simulink model "mcb_bldc_sixstep_f28069mLaunchPad_openLoop"  (R2023b)
settings: Solver=FixedStepDiscrete  StartTime=0.0  StopTime=2  RelTol=1e-3  EnableMultiTasking=on
InitFcn:
  | mcb_bldc_sixstep_f28069mLaunchPad_data;
undefined symbols (not defined in the file): bldc, Down, GPTRIP1SEL, GPTRIP2SEL, target, TZ1, TZ2, Up
libraries: c2806xlib x4, c2802xlib x4, mcbpositiondecoderlib x3, mcbcontrolslib x2, c280xlib x2, simulink x1, svdschedulerlib x1
settings Model: SILPILSystemUnderTest=refmodels  ExtModeTrigDuration=8  VariantFading=off  Creator=The MathWorks, Inc.  LastModifiedBy=Tefilus
settings SolverCC: AlgebraicLoopSolver=TrustRegion  AutoInsertRateTranBlk=on
settings DataIOCC: LimitDataPoints=on  SaveFormat=Array  SaveOutput=off  SaveTime=off  ReturnWorkspaceOutputs=off
settings OptimizationCC: DefaultParameterBehavior=Inlined  DefaultUnderspecifiedDataType=single  OptimizeBlockIOStorage=off  BufferReuse=off  ReuseModelBlockBuffer=off  GlobalBufferReuse=off  ExpressionFolding=off  ExpressionDepthLimit=2147483647  LocalBlockOutputs=off  InitFltsAndDblsToZero=on  NoFixptDivByZeroProtection=on  EfficientFloat2IntCast=on  EfficientMapNaN2IntZero=off  LifeSpan=inf  MaxStackSize=1024  OptimizeDataStoreBuffers=off  BusAssignmentInplaceUpdate=off  DenormalBehavior=FlushToZero  EfficientTunableParamExpr=on
settings DebuggingCC: AlgebraicLoopMsg=error  ArtificialAlgebraicLoopMsg=error  CheckSSInitialOutputMsg=off  MergeDetectMultiDrivingBlocksExec=none  SolverPrmCheckMsg=warning  InheritedTsInSrcMsg=none  MultiTaskDSMMsg=none  MultiTaskCondExecSysMsg=none  TasksWithSamePriorityMsg=none  SigSpecEnsureSampleTimeMsg=none  ParameterPrecisionLossMsg=none  ParameterTunabilityLossMsg=error  FcnCallInpInsideContextMsg=warning  UnconnectedInputMsg=warning  UnconnectedOutputMsg=warning  UnconnectedLineMsg=warning  AllowSymbolicDim=off  StateNameClashWarn=warning  SFUnexpectedBacktrackingDiag=warning  SFNoUnconditionalDefaultTransitionDiag=warning  SFExecutionAtInitializationDiag=none  ArithmeticOperatorsInVariantConditions=warning
settings HardwareCC: ProdBitPerChar=16  ProdBitPerInt=16  ProdBitPerPointer=32  ProdBitPerSizeT=32  ProdBitPerPtrDiffT=32  ProdLargestAtomicInteger=Integer  ProdLargestAtomicFloat=None  ProdWordSize=16  ProdLongLongMode=on  ProdHWDeviceType=Texas Instruments->C2000  TargetBitPerChar=16  TargetBitPerInt=16  TargetLargestAtomicInteger=Integer  TargetLongLongMode=on  TargetIntDivRoundTo=Zero  TargetEndianess=LittleEndian  TargetWordSize=16  TargetHWDeviceType=Texas Instruments->C2000  ProdEqTarget=off
settings ModelReferenceCC: EnableRefExpFcnMdlSchedulingChecks=on  PropagateSignalLabelsOutOfModel=off
settings SFSimCC: SimUseLocalCustomCode=off  MATLABDynamicMemAlloc=off
settings RTWCC: Description=Embedded Coder  SystemTargetFile=ert.tlc  HardwareBoard=TI Piccolo F28069M LaunchPad  TemplateMakefile=ert_default_tmf  PostCodeGenCommand=; codertarget.postCodeGenHookCommand(h)  GenerateReport=on  RTWUseLocalCustomCode=off  Toolchain=Texas Instruments Code Composer Studio (C2000)  IncludeHyperlinkInReport=on  GenerateTraceInfo=on  GenerateTraceReport=on  GenerateTraceReportSl=on  GenerateTraceReportSf=on  GenerateTraceReportEml=on  DLArmComputeVersion=19.05
settings CodeAppCC: IgnoreCustomStorageClasses=off  CustomSymbolStrType=$N$R$M  StateflowObjectComments=on  InternalIdentifier=Classic
settings ERTTargetCC: TargetFcnLib=ansi_tfl_tmw_new.mat  CodeReplacementLibrary=TI C28x  MultiwordLength=2048  ParMdlRefBuildCompliant=off  CompOptLevelCompliant=off  ConcurrentExecutionCompliant=off  CPPClassGenCompliant=off  ExtModeStaticAllocSize=2000  ExtModeMexFile=TIC2000ExternalModeOpen  ExtModeIntrfLevel=Level2 - Open  ConvertIfToSwitch=off  SuppressUnreachableDefaultCases=off  MemSecPackage=tic2000demospkg
settings ConfigComp: CovMetricSettings=dw  CovSaveCumulativeToWorkspaceVar=on  CovSaveSingleToWorkspaceVar=on  CovExternalEMLEnable=off  CovSFcnEnable=off

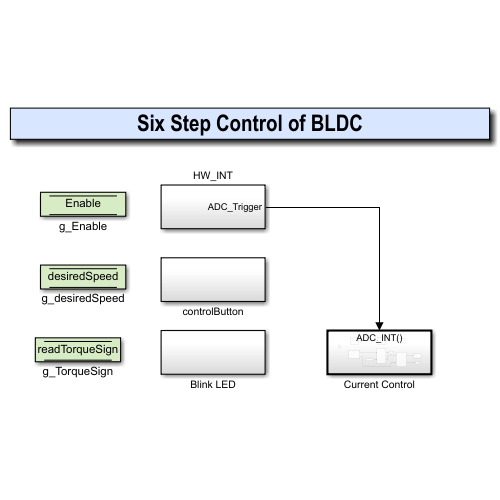
[thumbnail: Simulink's stored preview of the top-level diagram]
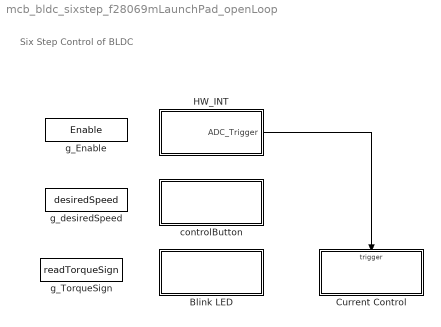
== system mcb_bldc_sixstep_f28069mLaunchPad_openLoop ==
  note: Six Step Control of BLDC
  Blink LED : Subsystem
  Current Control : Subsystem  TreatAsAtomicUnit=on
  HW_INT : Subsystem
  controlButton : Subsystem
  g_Enable : DataStoreMemory  DataStoreName=Enable  ShowAdditionalParam=off  OutDataTypeStr=boolean
  g_TorqueSign : DataStoreMemory  DataStoreName=readTorqueSign  ShowAdditionalParam=off  OutDataTypeStr=boolean
  g_desiredSpeed : DataStoreMemory  DataStoreName=desiredSpeed  ShowAdditionalParam=off
  wires:
  HW_INT/1(ADC_Trigger) -> Current Control/Trigger

== system mcb_bldc_sixstep_f28069mLaunchPad_openLoop/Blink LED ==
  Constant : Constant  SampleTime=0.5
  Digital Output : c2806xlib/Digital Output  GPIO_Number=GPIO32~GPIO39  GPIO_Bit0=off  GPIO_BIT0_Toggle=off  GPIO_Bit1=off  GPIO_BIT1_Toggle=off  GPIO_Bit2=off  GPIO_BIT2_Toggle=off  GPIO_Bit3=off  GPIO_BIT3_Toggle=off  GPIO_Bit4=off  GPIO_BIT4_Toggle=off  GPIO_Bit5=off  GPIO_BIT5_Toggle=off  GPIO_Bit6=off  GPIO_BIT6_Toggle=off  GPIO_Bit7=on  GPIO_BIT7_Toggle=on
  wires:
  Constant/1 -> Digital Output/1

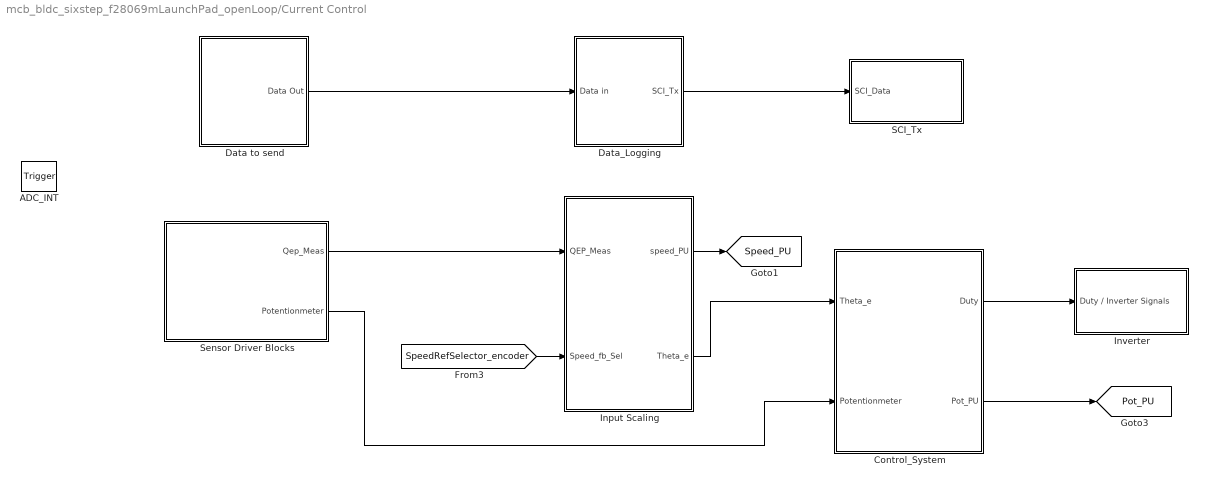
== system mcb_bldc_sixstep_f28069mLaunchPad_openLoop/Current Control ==
  ADC_INT : TriggerPort  TriggerType=function-call  VariantControl=(inherit)
  Control_System : Subsystem
  Data to send : Subsystem
  Data_Logging : Subsystem
  Input Scaling : Subsystem
  Inverter : Subsystem  VariantControl=(codegen)
  SCI_Tx : Subsystem  VariantControl=(codegen)
  Sensor Driver Blocks : Subsystem  VariantControl=(codegen)
  tag scope: Pot_PU=global, Speed_PU=global
  wires:
  Control_System/1(Duty) -> Inverter/1(Duty / Inverter Signals)
  Input Scaling/2(Theta_e) -> Control_System/1(Theta_e)
  Sensor Driver Blocks/2(Potentionmeter) -> Control_System/2(Potentionmeter)
  Data_Logging/1(SCI_Tx) -> SCI_Tx/1(SCI_Data)
  Control_System/2(Pot_PU) -> [Pot_PU]
  Input Scaling/1(speed_PU) -> [Speed_PU]
  [SpeedRefSelector_encoder] -> Input Scaling/2(Speed_fb_Sel)
  Data to send/1(Data Out) -> Data_Logging/1(Data in)
  Sensor Driver Blocks/1(Qep_Meas) -> Input Scaling/1(QEP_Meas)

== system mcb_bldc_sixstep_f28069mLaunchPad_openLoop/HW_INT ==
  HWI_ADCINT1 : svdschedulerlib/Hardware Interrupt v2  ISRGroup=ADC - Analog to Digital Converter  ISRName=ADCA1_INT  ISRNumber=32  NumEventsToServe=1  EventsList={'on','EOC event','1';'off','Overflow event','2';'off','Custom event','3'}  SelectedEvents={'event1'}  TaskPriority=30  DisablePreemption=on  ClearInterruptFlagsAtEndOfEvent=on  InterruptDefinitionFile=$(TARGET_ROOT)/registry/interrupts/F2837xS_interrupts.xml  HardwareBoard=F2837x  EnableSimPort=off
      settings: LibrarySourceBlock=c2000lib/Scheduling/Hardware Interrupt
  ADC_Trigger : Outport
  wires:
  HWI_ADCINT1/1 -> ADC_Trigger/1

== system mcb_bldc_sixstep_f28069mLaunchPad_openLoop/controlButton ==
  CW/CCW_GPIO7 : c2806xlib/Digital Input  GPIO_Number=GPIO0~GPIO7  GPIO_Bit0=off  GPIO_Bit1=off  GPIO_Bit2=off  GPIO_Bit3=off  GPIO_Bit4=off  GPIO_Bit5=off  GPIO_Bit6=off  GPIO_Bit7=on  sampleTime=0.1  dataType=auto  GPIO_Bit0_Qualification=Sync to SYSCLKOUT  GPIO_Bit1_Qualification=Sync to SYSCLKOUT  GPIO_Bit2_Qualification=Sync to SYSCLKOUT  GPIO_Bit3_Qualification=Sync to SYSCLKOUT  GPIO_Bit4_Qualification=Sync to SYSCLKOUT  GPIO_Bit5_Qualification=Sync to SYSCLKOUT  GPIO_Bit6_Qualification=Sync to SYSCLKOUT  GPIO_Bit7_Qualification=Sync to SYSCLKOUT  Qualification_Period=-1
  Data Store Write : DataStoreWrite  DataStoreName=Enable  IndexOptions=Index vector (dialog)  Indices=1  OutputSizes=1
  Data Store Write1 : DataStoreWrite  DataStoreName=readTorqueSign  IndexOptions=Index vector (dialog)  Indices=1  OutputSizes=1
  ON/OFF_GPIO6 : c2806xlib/Digital Input  GPIO_Number=GPIO0~GPIO7  GPIO_Bit0=off  GPIO_Bit1=off  GPIO_Bit2=off  GPIO_Bit3=off  GPIO_Bit4=off  GPIO_Bit5=off  GPIO_Bit6=on  GPIO_Bit7=off  sampleTime=0.1  dataType=auto  GPIO_Bit0_Qualification=Sync to SYSCLKOUT  GPIO_Bit1_Qualification=Sync to SYSCLKOUT  GPIO_Bit2_Qualification=Sync to SYSCLKOUT  GPIO_Bit3_Qualification=Sync to SYSCLKOUT  GPIO_Bit4_Qualification=Sync to SYSCLKOUT  GPIO_Bit5_Qualification=Sync to SYSCLKOUT  GPIO_Bit6_Qualification=Sync to SYSCLKOUT  GPIO_Bit7_Qualification=Sync to SYSCLKOUT  Qualification_Period=-1
  wires:
  ON/OFF_GPIO6/1 -> Data Store Write/1
  CW/CCW_GPIO7/1 -> Data Store Write1/1

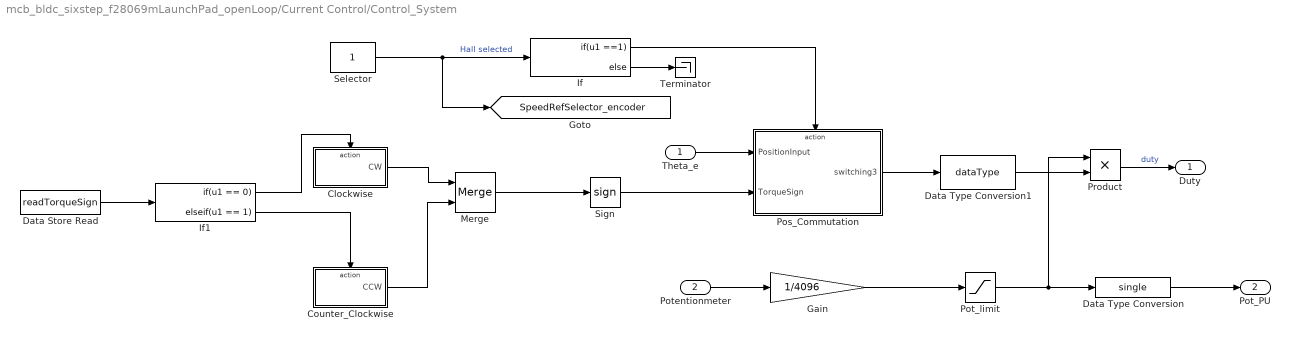
== system mcb_bldc_sixstep_f28069mLaunchPad_openLoop/Current Control/Control_System ==
  Theta_e : Inport
  Potentionmeter : Inport  Port=2
  Clockwise : Subsystem  TreatAsAtomicUnit=on
  Counter_Clockwise : Subsystem  TreatAsAtomicUnit=on
  Data Store Read : DataStoreRead  DataStoreName=readTorqueSign  IndexOptions=Index vector (dialog)  Indices=1  OutputSizes=1
  Data Type Conversion : DataTypeConversion  OutDataTypeStr=single  SaturateOnIntegerOverflow=off  RndMeth=Floor
  Data Type Conversion1 : DataTypeConversion  OutDataTypeStr=dataType  RndMeth=Simplest  SaturateOnIntegerOverflow=off
  Gain : Gain  Gain=1/4096
  If : If  IfExpression=u1 ==1
  If1 : If  IfExpression=u1 == 0  ElseIfExpressions=u1 == 1  ShowElse=off
  Merge : Merge
  Pos_Commutation : Subsystem
  Pot_limit : Saturate  UpperLimit=0.9  LowerLimit=0
  Product : Product  RndMeth=Simplest  OutDataTypeStr=Inherit: Same as first input
  Selector : Constant  OutDataTypeStr=uint16  SampleTime=-1
  Sign : Signum
  Terminator : Terminator
  Duty : Outport  VectorParamsAs1DForOutWhenUnconnected=off
  Pot_PU : Outport  Port=2
  tag scope: SpeedRefSelector_encoder=global
  wires:
  If/1 -> Pos_Commutation/Action
  Pos_Commutation/1(switching3) -> Data Type Conversion1/1
  Product/1 -> Duty/1  "duty"
  Selector/1 -> If/1, [SpeedRefSelector_encoder]  "Hall selected"
  If/2 -> Terminator/1
  Data Store Read/1 -> If1/1
  If1/1 -> Clockwise/Action
  Clockwise/1(CW) -> Merge/1
  Counter_Clockwise/1(CCW) -> Merge/2
  Merge/1 -> Sign/1
  If1/2 -> Counter_Clockwise/Action
  Pot_limit/1 -> Product/1, Data Type Conversion/1
  Data Type Conversion1/1 -> Product/2
  Data Type Conversion/1 -> Pot_PU/1
  Sign/1 -> Pos_Commutation/2(TorqueSign)
  Theta_e/1 -> Pos_Commutation/1(PositionInput)
  Potentionmeter/1 -> Gain/1
  Gain/1 -> Pot_limit/1

== system mcb_bldc_sixstep_f28069mLaunchPad_openLoop/Current Control/Data to send ==
  Mux : Mux  Inputs=2
  Data Out : Outport
  wires:
  [Speed_PU] -> Mux/1
  Mux/1 -> Data Out/1
  [Pot_PU] -> Mux/2

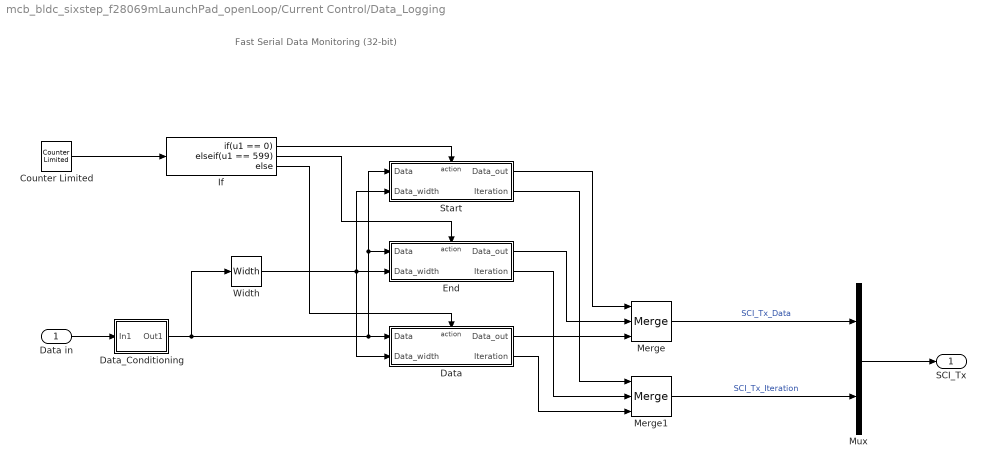
== system mcb_bldc_sixstep_f28069mLaunchPad_openLoop/Current Control/Data_Logging ==
  note: Fast Serial Data Monitoring (32-bit)
  Data in : Inport
  Counter Limited : simulink/Sources/Counter Limited  uplimit=599  tsamp=-1
  Data : Subsystem  TreatAsAtomicUnit=on
  Data_Conditioning : Subsystem
  End : Subsystem  TreatAsAtomicUnit=on
  If : If  IfExpression=u1 == 0  ElseIfExpressions=u1 == 599
  Merge : Merge  Inputs=3
  Merge1 : Merge  Inputs=3
  Mux : Mux  Inputs=2
  Start : Subsystem  TreatAsAtomicUnit=on
  Width : Width  OutDataTypeMode=All ports same datatype  DataType=uint16
  SCI_Tx : Outport
  wires:
  If/3 -> Data/Action
  Data/1(Data_out) -> Merge/3
  Width/1 -> Data/2(Data_width), Start/2(Data_width), End/2(Data_width)
  Merge/1 -> Mux/1  "SCI_Tx_Data"
  Counter Limited/1 -> If/1
  Start/2(Iteration) -> Merge1/1
  Start/1(Data_out) -> Merge/1
  If/2 -> End/Action
  Merge1/1 -> Mux/2  "SCI_Tx_Iteration"
  If/1 -> Start/Action
  End/1(Data_out) -> Merge/2
  End/2(Iteration) -> Merge1/2
  Data/2(Iteration) -> Merge1/3
  Data_Conditioning/1(Out1) -> Width/1, Start/1(Data), End/1(Data), Data/1(Data)
  Mux/1 -> SCI_Tx/1
  Data in/1 -> Data_Conditioning/1(In1)

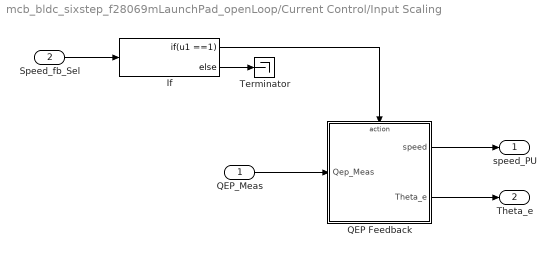
== system mcb_bldc_sixstep_f28069mLaunchPad_openLoop/Current Control/Input Scaling ==
  QEP_Meas : Inport
  Speed_fb_Sel : Inport  Port=2
  If : If  IfExpression=u1 ==1
  QEP Feedback : Subsystem  TreatAsAtomicUnit=on
  Terminator : Terminator
  speed_PU : Outport  InitialOutput=0  VectorParamsAs1DForOutWhenUnconnected=off
  Theta_e : Outport  Port=2  InitialOutput=0  VectorParamsAs1DForOutWhenUnconnected=off
  wires:
  Speed_fb_Sel/1 -> If/1
  QEP_Meas/1 -> QEP Feedback/1(Qep_Meas)
  If/1 -> QEP Feedback/Action
  QEP Feedback/1(speed) -> speed_PU/1
  If/2 -> Terminator/1
  QEP Feedback/2(Theta_e) -> Theta_e/1

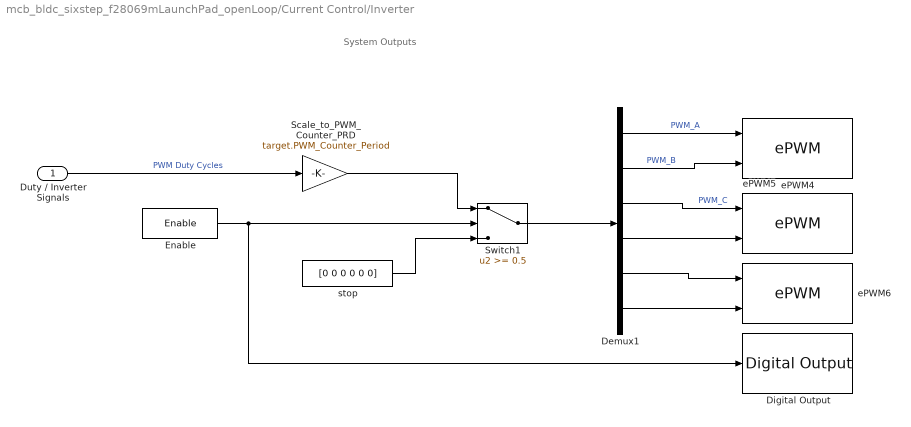
== system mcb_bldc_sixstep_f28069mLaunchPad_openLoop/Current Control/Inverter ==
  note: System Outputs
  Duty / Inverter Signals : Inport
  Demux1 : Demux  Outputs=6
  Digital Output : c2806xlib/Digital Output  GPIO_Number=GPIO8~GPIO15  GPIO_Bit0=off  GPIO_BIT0_Toggle=off  GPIO_Bit1=off  GPIO_BIT1_Toggle=off  GPIO_Bit2=off  GPIO_BIT2_Toggle=off  GPIO_Bit3=off  GPIO_BIT3_Toggle=off  GPIO_Bit4=off  GPIO_BIT4_Toggle=off  GPIO_Bit5=on  GPIO_BIT5_Toggle=off  GPIO_Bit6=off  GPIO_BIT6_Toggle=off  GPIO_Bit7=off  GPIO_BIT7_Toggle=off
  Enable : DataStoreRead  DataStoreName=Enable  IndexOptions=Index vector (dialog)  Indices=1  OutputSizes=1
  Scale_to_PWM_Counter_PRD : Gain  Gain=target.PWM_Counter_Period  OutDataTypeStr=uint16  RndMeth=Simplest
  Switch1 : Switch  Threshold=0.5  SaturateOnIntegerOverflow=off  InputSameDT=off
  ePWM4 : c2802xlib/ePWM  PwmType=C2000  useModule=ePWM1  ePWMxLINKTBPRD=Not Linked  periodUnits=Clock cycles  timerSource=Specify via dialog  timerPeriod_clk=target.PWM_Counter_Period  timerPeriod_sec=64000  tbshadow=Counter equals to zero  countingMode=Up-Down  phaseActiveEnable=Disable  phaseDirection=Count down after sync  phaseActive=0  synchronizationEnable=off  dcaevt1Sync=off  dcbevt1Sync=off  synchronizationOption=Counter equals to zero (CTR=Zero)  dcbevt1SyncOut=off  dcaevt1SyncOut=off  cmpdSyncOut=off  cmpcSyncOut=off  cmpbSyncOut=off  zeroSyncOut=on  swfSyncOut=off  perSynchronizationOption=Counter equals to period (CTR=PRD)  clockPrescale=1  HSclockPrescale=1  enswap=off  ePWMxAStatus=on  ePWMxAactionLogic1=Do nothing  ePWMxAactionLogic2=Do nothing  ePWMxAactionLogic3=Clear  ePWMxAactionLogic4=Set  ePWMxAactionLogic5=Do nothing  ePWMxAactionLogic6=Do nothing  ePWMxACSFenable=off  ePWMxACSFvalue=Forcing disable  ePWMxASFreload=Zero  ePWMxBStatus=on  ePWMxBactionLogic1=Do nothing  ePWMxBactionLogic2=Do nothing  ePWMxBactionLogic3=Do nothing  ePWMxBactionLogic4=Do nothing  ePWMxBactionLogic5=Clear  ePWMxBactionLogic6=Set  ePWMxBCSFenable=off  ePWMxBCSFvalue=Forcing disable  ePWMxBSFreload=Zero  ePWNxBOutWay=off  ePWMxLINKCMPA=Not Linked  CMPAUnits=Clock cycles  CMPASource=Input port  CMPAValue_per=32000  CMPAValue_clk=floor(target.PWM_Counter_Period/2+1)  enCMPAshadow=Counter equals to zero (CTR=Zero)  ePWMxLINKCMPB=Not Linked  CMPBUnits=Clock cycles  CMPBSource=Input port  CMPBValue_per=50  CMPBValue_clk=floor(target.PWM_Counter_Period/2+1)  enCMPBshadow=Counter equals to zero (CTR=Zero)  ePWMxLINKCMPC=Not Linked  CMPCUnits=Clock cycles  CMPCSource=Specify via dialog  CMPCValue_per=50  CMPCValue_clk=32000  enCMPCshadow=Counter equals to zero (CTR=Zero)  ePWMxLINKCMPD=Not Linked  CMPDUnits=Clock cycles  CMPDSource=Specify via dialog  CMPDValue_per=50  CMPDValue_clk=32000  enCMPDshadow=Counter equals to zero (CTR=Zero)  enableDBePWMxA=off  enableDBePWMxB=off  enhalfcycle=off  DBpolarity=Active high complementary (AHC)  DBedgeDelay=Positive  DBSource_ePWMxA=ePWMxA  DBSource_ePWMxB=ePWMxA  DBPeriodUnits=Clock cycles  DBperiodSource=Specify via dialog  REDperiod=15  FEDperiod=15  REDperiod_sec=0  FEDperiod_sec=0  LoadModeDBRED=Immediate without using shadow  LoadModeDBFED=Immediate without using shadow  adcstartModuleA=on  adcrequestEventA=First event  adcstartEventA=Counter equals to zero (CTR=Zero)  adcstartEventA_type2=Digital Compare Module A Event 1 start of conversion (DCAEVT1.soc)  adcstartModuleB=on  adcrequestEventB=First event  adcstartEventB=Counter equals to zero (CTR=Zero)  adcstartEventB_type2=Counter equals to zero (CTR=Zero)  intEn=off  intPrd=First event  intSel=Counter equals to zero (CTR=Zero)  intSel_type2=Counter equals to zero (CTR=Zero)  hrpe=off  enHRPWM=off  HRPWM_LoadMode=Counter equals to period (CTR=PRD)  HRPWM_CTLMode=Duty or Period control mode  HRPWM_EDGMode=Both edge  hrpeb=off  enHRPWMB=off  HRPWM_LoadModeB=Counter equals to zero (CTR=ZERO)  HRPWM_CTLModeB=Duty or Period control mode  HRPWM_EDGModeB=Both edge  enHRDBRED=off  enHRDBFED=off  enSFO=on  enautoconv=on  chopperEnable=off  chopperFrequency=1  chopperFirstwidth=1  chopperDuty=12.5%  tripZonesource=Specify via dialog  tzselOSHT1=off  tzselOSHT2=off  tzselOSHT3=off  tzselOSHDCAEV1=off  tzselOSHDCBEV1=off  tzselCBC1=off  tzselCBC2=off  tzselCBC3=off  tzselCBCDCAEV2=off  tzselCBCDCBEV2=off  tzselOSHT4=off  tzselOSHT5=off  tzselOSHT6=off  tzselCBC4=off  tzselCBC5=off  tzselCBC6=off  enTzOstIntr=off  enTzCbcIntr=off  enTzDCAEVT1Intr=off  enTzDCAEVT2Intr=off  enTzDCBEVT1Intr=off  enTzDCBEVT2Intr=off  ePWMxAforced=No action  ePWMxBforced=No action  DCAEVT1forced=No action  DCBEVT1forced=No action  DCAEVT2forced=No action  DCBEVT2forced=No action  dcah=Trip Zone 1 input (TZ1)  dcal=Trip Zone 2 input (TZ2)  dcbh=Trip Zone 1 input (TZ1)  dcbl=Trip Zone 2 input (TZ2)  dcah_type2=GPTRIP1SEL/(TZ1)  dcal_type2=GPTRIP2SEL/(TZ2)  dcbh_type2=GPTRIP1SEL/(TZ1)  dcbl_type2=GPTRIP2SEL/(TZ2)  gendcaevt1=Event disabled  gendcaevt2=Event disabled  gendcbevt1=Event disabled  gendcbevt2=Event disabled  dcaevt1src=DCAEVT1 with sync  dcaevt2src=DCAEVT2 with sync  dcbevt1src=DCBEVT1 with sync  dcbevt2src=DCBEVT2 with sync  pulsesel=Counter equals to zero (CTR=Zero)  blankinv=off  blankoffset=0  blankwidth=0  evsrcsel=Filtered version of DCAEVT1 (DCAEVT1FILT)  encape=off
  ePWM5 : c2802xlib/ePWM  PwmType=C2000  useModule=ePWM2  ePWMxLINKTBPRD=Not Linked  periodUnits=Clock cycles  timerSource=Specify via dialog  timerPeriod_clk=target.PWM_Counter_Period  timerPeriod_sec=64000  tbshadow=Counter equals to zero  countingMode=Up-Down  phaseActiveEnable=Set counter to phase value specified via dialog  phaseDirection=Count up after sync  phaseActive=0  synchronizationEnable=off  dcaevt1Sync=off  dcbevt1Sync=off  synchronizationOption=Pass through (EPWMxSYNCI or SWFSYNC)  dcbevt1SyncOut=off  dcaevt1SyncOut=off  cmpdSyncOut=off  cmpcSyncOut=off  cmpbSyncOut=off  zeroSyncOut=off  swfSyncOut=on  perSynchronizationOption=Counter equals to period (CTR=PRD)  clockPrescale=1  HSclockPrescale=1  enswap=off  ePWMxAStatus=on  ePWMxAactionLogic1=Do nothing  ePWMxAactionLogic2=Do nothing  ePWMxAactionLogic3=Clear  ePWMxAactionLogic4=Set  ePWMxAactionLogic5=Do nothing  ePWMxAactionLogic6=Do nothing  ePWMxACSFenable=off  ePWMxACSFvalue=Forcing disable  ePWMxASFreload=Zero  ePWMxBStatus=on  ePWMxBactionLogic1=Do nothing  ePWMxBactionLogic2=Do nothing  ePWMxBactionLogic3=Do nothing  ePWMxBactionLogic4=Do nothing  ePWMxBactionLogic5=Clear  ePWMxBactionLogic6=Set  ePWMxBCSFenable=off  ePWMxBCSFvalue=Forcing disable  ePWMxBSFreload=Zero  ePWNxBOutWay=off  ePWMxLINKCMPA=Not Linked  CMPAUnits=Clock cycles  CMPASource=Input port  CMPAValue_per=32000  CMPAValue_clk=floor(target.PWM_Counter_Period/2+1)  enCMPAshadow=Counter equals to zero (CTR=Zero)  ePWMxLINKCMPB=Not Linked  CMPBUnits=Clock cycles  CMPBSource=Input port  CMPBValue_per=50  CMPBValue_clk=floor(target.PWM_Counter_Period/2+1)  enCMPBshadow=Counter equals to zero (CTR=Zero)  ePWMxLINKCMPC=Not Linked  CMPCUnits=Clock cycles  CMPCSource=Specify via dialog  CMPCValue_per=50  CMPCValue_clk=32000  enCMPCshadow=Counter equals to zero (CTR=Zero)  ePWMxLINKCMPD=Not Linked  CMPDUnits=Clock cycles  CMPDSource=Specify via dialog  CMPDValue_per=50  CMPDValue_clk=32000  enCMPDshadow=Counter equals to zero (CTR=Zero)  enableDBePWMxA=off  enableDBePWMxB=off  enhalfcycle=off  DBpolarity=Active high complementary (AHC)  DBedgeDelay=Positive  DBSource_ePWMxA=ePWMxA  DBSource_ePWMxB=ePWMxA  DBPeriodUnits=Clock cycles  DBperiodSource=Specify via dialog  REDperiod=15  FEDperiod=15  REDperiod_sec=0  FEDperiod_sec=0  LoadModeDBRED=Immediate without using shadow  LoadModeDBFED=Immediate without using shadow  adcstartModuleA=off  adcrequestEventA=First event  adcstartEventA=Digital Compare Module A Event 1 start of conversion (DCAEVT1.soc)  adcstartEventA_type2=Digital Compare Module A Event 1 start of conversion (DCAEVT1.soc)  adcstartModuleB=off  adcrequestEventB=First event  adcstartEventB=Counter equals to zero (CTR=Zero)  adcstartEventB_type2=Counter equals to zero (CTR=Zero)  intEn=off  intPrd=First event  intSel=Counter equals to zero (CTR=Zero)  intSel_type2=Counter equals to zero (CTR=Zero)  hrpe=off  enHRPWM=off  HRPWM_LoadMode=Counter equals to period (CTR=PRD)  HRPWM_CTLMode=Duty or Period control mode  HRPWM_EDGMode=Both edge  hrpeb=off  enHRPWMB=off  HRPWM_LoadModeB=Counter equals to zero (CTR=ZERO)  HRPWM_CTLModeB=Duty or Period control mode  HRPWM_EDGModeB=Both edge  enHRDBRED=off  enHRDBFED=off  enSFO=on  enautoconv=on  chopperEnable=off  chopperFrequency=1  chopperFirstwidth=1  chopperDuty=12.5%  tripZonesource=Specify via dialog  tzselOSHT1=off  tzselOSHT2=off  tzselOSHT3=off  tzselOSHDCAEV1=off  tzselOSHDCBEV1=off  tzselCBC1=off  tzselCBC2=off  tzselCBC3=off  tzselCBCDCAEV2=off  tzselCBCDCBEV2=off  tzselOSHT4=off  tzselOSHT5=off  tzselOSHT6=off  tzselCBC4=off  tzselCBC5=off  tzselCBC6=off  enTzOstIntr=off  enTzCbcIntr=off  enTzDCAEVT1Intr=off  enTzDCAEVT2Intr=off  enTzDCBEVT1Intr=off  enTzDCBEVT2Intr=off  ePWMxAforced=No action  ePWMxBforced=No action  DCAEVT1forced=No action  DCBEVT1forced=No action  DCAEVT2forced=No action  DCBEVT2forced=No action  dcah=Trip Zone 1 input (TZ1)  dcal=Trip Zone 2 input (TZ2)  dcbh=Trip Zone 1 input (TZ1)  dcbl=Trip Zone 2 input (TZ2)  dcah_type2=GPTRIP1SEL/(TZ1)  dcal_type2=GPTRIP2SEL/(TZ2)  dcbh_type2=GPTRIP1SEL/(TZ1)  dcbl_type2=GPTRIP2SEL/(TZ2)  gendcaevt1=Event disabled  gendcaevt2=Event disabled  gendcbevt1=Event disabled  gendcbevt2=Event disabled  dcaevt1src=DCAEVT1 with sync  dcaevt2src=DCAEVT2 with sync  dcbevt1src=DCBEVT1 with sync  dcbevt2src=DCBEVT2 with sync  pulsesel=Counter equals to zero (CTR=Zero)  blankinv=off  blankoffset=0  blankwidth=0  evsrcsel=Filtered version of DCAEVT1 (DCAEVT1FILT)  encape=off
  ePWM6 : c2802xlib/ePWM  PwmType=C2000  useModule=ePWM3  ePWMxLINKTBPRD=Not Linked  periodUnits=Clock cycles  timerSource=Specify via dialog  timerPeriod_clk=target.PWM_Counter_Period  timerPeriod_sec=64000  tbshadow=Counter equals to zero  countingMode=Up-Down  phaseActiveEnable=Set counter to phase value specified via dialog  phaseDirection=Count up after sync  phaseActive=0  synchronizationEnable=off  dcaevt1Sync=off  dcbevt1Sync=off  synchronizationOption=Disable  dcbevt1SyncOut=off  dcaevt1SyncOut=off  cmpdSyncOut=off  cmpcSyncOut=off  cmpbSyncOut=off  zeroSyncOut=off  swfSyncOut=off  perSynchronizationOption=Counter equals to period (CTR=PRD)  clockPrescale=1  HSclockPrescale=1  enswap=off  ePWMxAStatus=on  ePWMxAactionLogic1=Do nothing  ePWMxAactionLogic2=Do nothing  ePWMxAactionLogic3=Clear  ePWMxAactionLogic4=Set  ePWMxAactionLogic5=Do nothing  ePWMxAactionLogic6=Do nothing  ePWMxACSFenable=off  ePWMxACSFvalue=Forcing disable  ePWMxASFreload=Zero  ePWMxBStatus=on  ePWMxBactionLogic1=Do nothing  ePWMxBactionLogic2=Do nothing  ePWMxBactionLogic3=Do nothing  ePWMxBactionLogic4=Do nothing  ePWMxBactionLogic5=Clear  ePWMxBactionLogic6=Set  ePWMxBCSFenable=off  ePWMxBCSFvalue=Forcing disable  ePWMxBSFreload=Zero  ePWNxBOutWay=off  ePWMxLINKCMPA=Not Linked  CMPAUnits=Clock cycles  CMPASource=Input port  CMPAValue_per=32000  CMPAValue_clk=floor(target.PWM_Counter_Period/2+1)  enCMPAshadow=Counter equals to zero (CTR=Zero)  ePWMxLINKCMPB=Not Linked  CMPBUnits=Clock cycles  CMPBSource=Input port  CMPBValue_per=50  CMPBValue_clk=floor(target.PWM_Counter_Period/2+1)  enCMPBshadow=Counter equals to zero (CTR=Zero)  ePWMxLINKCMPC=Not Linked  CMPCUnits=Clock cycles  CMPCSource=Specify via dialog  CMPCValue_per=50  CMPCValue_clk=32000  enCMPCshadow=Counter equals to zero (CTR=Zero)  ePWMxLINKCMPD=Not Linked  CMPDUnits=Clock cycles  CMPDSource=Specify via dialog  CMPDValue_per=50  CMPDValue_clk=32000  enCMPDshadow=Counter equals to zero (CTR=Zero)  enableDBePWMxA=off  enableDBePWMxB=off  enhalfcycle=off  DBpolarity=Active high complementary (AHC)  DBedgeDelay=Positive  DBSource_ePWMxA=ePWMxA  DBSource_ePWMxB=ePWMxA  DBPeriodUnits=Clock cycles  DBperiodSource=Specify via dialog  REDperiod=15  FEDperiod=15  REDperiod_sec=0  FEDperiod_sec=0  LoadModeDBRED=Immediate without using shadow  LoadModeDBFED=Immediate without using shadow  adcstartModuleA=off  adcrequestEventA=First event  adcstartEventA=Digital Compare Module A Event 1 start of conversion (DCAEVT1.soc)  adcstartEventA_type2=Digital Compare Module A Event 1 start of conversion (DCAEVT1.soc)  adcstartModuleB=off  adcrequestEventB=First event  adcstartEventB=Counter equals to zero (CTR=Zero)  adcstartEventB_type2=Counter equals to zero (CTR=Zero)  intEn=off  intPrd=First event  intSel=Counter equals to zero (CTR=Zero)  intSel_type2=Counter equals to zero (CTR=Zero)  hrpe=off  enHRPWM=off  HRPWM_LoadMode=Counter equals to period (CTR=PRD)  HRPWM_CTLMode=Duty or Period control mode  HRPWM_EDGMode=Both edge  hrpeb=off  enHRPWMB=off  HRPWM_LoadModeB=Counter equals to zero (CTR=ZERO)  HRPWM_CTLModeB=Duty or Period control mode  HRPWM_EDGModeB=Both edge  enHRDBRED=off  enHRDBFED=off  enSFO=on  enautoconv=on  chopperEnable=off  chopperFrequency=1  chopperFirstwidth=1  chopperDuty=12.5%  tripZonesource=Specify via dialog  tzselOSHT1=off  tzselOSHT2=off  tzselOSHT3=off  tzselOSHDCAEV1=off  tzselOSHDCBEV1=off  tzselCBC1=off  tzselCBC2=off  tzselCBC3=off  tzselCBCDCAEV2=off  tzselCBCDCBEV2=off  tzselOSHT4=off  tzselOSHT5=off  tzselOSHT6=off  tzselCBC4=off  tzselCBC5=off  tzselCBC6=off  enTzOstIntr=off  enTzCbcIntr=off  enTzDCAEVT1Intr=off  enTzDCAEVT2Intr=off  enTzDCBEVT1Intr=off  enTzDCBEVT2Intr=off  ePWMxAforced=No action  ePWMxBforced=No action  DCAEVT1forced=No action  DCBEVT1forced=No action  DCAEVT2forced=No action  DCBEVT2forced=No action  dcah=Trip Zone 1 input (TZ1)  dcal=Trip Zone 2 input (TZ2)  dcbh=Trip Zone 1 input (TZ1)  dcbl=Trip Zone 2 input (TZ2)  dcah_type2=GPTRIP1SEL/(TZ1)  dcal_type2=GPTRIP2SEL/(TZ2)  dcbh_type2=GPTRIP1SEL/(TZ1)  dcbl_type2=GPTRIP2SEL/(TZ2)  gendcaevt1=Event disabled  gendcaevt2=Event disabled  gendcbevt1=Event disabled  gendcbevt2=Event disabled  dcaevt1src=DCAEVT1 with sync  dcaevt2src=DCAEVT2 with sync  dcbevt1src=DCBEVT1 with sync  dcbevt2src=DCBEVT2 with sync  pulsesel=Counter equals to zero (CTR=Zero)  blankinv=off  blankoffset=0  blankwidth=0  evsrcsel=Filtered version of DCAEVT1 (DCAEVT1FILT)  encape=off
  stop : Constant  Value=[0 0 0 0 0 0]  OutDataTypeStr=uint16
  wires:
  Scale_to_PWM_Counter_PRD/1 -> Switch1/1
  stop/1 -> Switch1/3
  Switch1/1 -> Demux1/1
  Duty / Inverter Signals/1 -> Scale_to_PWM_Counter_PRD/1  "PWM Duty Cycles"
  Enable/1 -> Digital Output/1, Switch1/2
  Demux1/1 -> ePWM4/1  "PWM_A"
  Demux1/2 -> ePWM4/2  "PWM_B"
  Demux1/3 -> ePWM5/1  "PWM_C"
  Demux1/4 -> ePWM5/2
  Demux1/5 -> ePWM6/1
  Demux1/6 -> ePWM6/2

== system mcb_bldc_sixstep_f28069mLaunchPad_openLoop/Current Control/SCI_Tx ==
  SCI_Data : Inport
  CodeGeneration : Subsystem  TreatAsAtomicUnit=on
  wires:
  SCI_Data/1 -> CodeGeneration/1(SCI_Data)

== system mcb_bldc_sixstep_f28069mLaunchPad_openLoop/Current Control/Sensor Driver Blocks ==
  Mux2 : Mux  Inputs=2
  Read POT : c2802xlib/ADC  blkParamProc=C2000  ADCModule=1  samplingMode=Single sample mode  ADCResolution=12-bit (Single-ended input)  useSOC1=SOC1  useSOC2=SOC0_SOC1  SOCAcquisitionWindow=7  SOCTriggerSource=ePWM1_ADCSOCA  SOCInterruptTrigger=No ADCINT  Ts=-1  dType=uint16  postInterrupt=on  interruptSel=ADCINT1  ADCINTContinuous=on  endma=off  chdma=1  conv1=ADCINB1  conv2=ADCINA0 and ADCINB0  conv1_Type4=ADCIN0  conv2_Type4=ADCIN0 and ADCIN1
      settings: LibrarySourceBlock=c2806xlib/ADC
  eQEP : c280xlib/eQEP  useModule=eQEP1  pcInputmode=Quadrature-count  externalClockrate=2x resolution: Count the rising/falling edge  swapPolarityselection=Clockwise  qdfOutputport=off  qapPolarityselection=on  qbpPolarityselection=on  qipPolarityselection=on  qspPolarityselection=off  igatePolarityselection=off  sampleTime=-1  pcOutputport=on  pcMaximumvalue=2^16-1  indexInitializationcheck=off  indexInitializationevent=Falling edge  strobeInitializationcheck=off  strobeInitializationevent=Rising edge  softwareInitializationcheck=off  softwareInitializationsource=Set to init value at start up  softwareInitializationmode=on  pcInitialvalue=0  pcResetmode=Reset on the first index event  ieloutputport=on  indexEventlatch=Falling edge  seloutputport=off  strobeEventlatch=Rising edge  pcefOutputport=off  enableEqepcapture=off  qctmrOutputport=off  qcprdOutputport=off  captureTimerprescaler=128  upEventprescaler=128  overflowErrorflag=off  directionErrorflag=off  captureTimerposition=On position counter read  unitTimerperiod=100000000  captureTimerlatch=off  capturePeriodlatch=off  positionCounterlatch=off  soenPolarityselection=off  spselPolarityselection=Index pin is used for sync output  compareValuesource=Specify via dialog  shadowMode=Load on QPOSCNT=0  compareValue=4294967295  syncOutputwidth=1  polaritySyncoutput=Active high  watchdogEnable=off  watchdogTimer=65535  outport1Datatype=auto  outport2Datatype=auto  outport3Datatype=auto  outport4Datatype=auto  outport5Datatype=auto  outport6Datatype=auto  outport7Datatype=auto  outport8Datatype=auto  outport9Datatype=auto  outport10Datatype=auto  outport11Datatype=auto  outport12Datatype=auto  eqepinterrupt_pce=off  eqepinterrupt_qpe=off  eqepinterrupt_qdc=off  eqepinterrupt_wto=off  eqepinterrupt_pcu=off  eqepinterrupt_pco=off  eqepinterrupt_pcr=off  eqepinterrupt_pcm=off  eqepinterrupt_sel=off  eqepinterrupt_iel=off  eqepinterrupt_uto=off  pheOutputport=off  watchdogOutputport=off  outport13Datatype=auto  outport14Datatype=auto
  Qep_Meas : Outport
  Potentionmeter : Outport  Port=2
  wires:
  Read POT/1 -> Potentionmeter/1
  eQEP/1 -> Mux2/1
  Mux2/1 -> Qep_Meas/1
  eQEP/2 -> Mux2/2

== system mcb_bldc_sixstep_f28069mLaunchPad_openLoop/Current Control/Control_System/Clockwise ==
  Action Port : ActionPort  ActionPortLabel=if(u1 == 0)
  Clockwise : Constant
  CW : Outport
  wires:
  Clockwise/1 -> CW/1

== system mcb_bldc_sixstep_f28069mLaunchPad_openLoop/Current Control/Control_System/Counter_Clockwise ==
  Action Port : ActionPort  ActionPortLabel=elseif(u1 == 1)
  Counter_Clockwise : Constant  Value=-1
  CCW : Outport
  wires:
  Counter_Clockwise/1 -> CCW/1

== system mcb_bldc_sixstep_f28069mLaunchPad_openLoop/Current Control/Control_System/Pos_Commutation ==
  PositionInput : Inport
  TorqueSign : Inport  Port=2
  Action Port : ActionPort  ActionPortLabel=if(u1 ==1)
  Six Step Commutation : mcbcontrolslib/Six Step Commutation  InputType=Position  PositionUnit=Per unit  CommutationMode=120 deg  SequencePos=[5,4,6,2,3,1]  EnableCustomSwitching=off  CommutationSeqPos=[1 0 0 1 0 0;1 0 0 0 0 1; 0 0 1 0 0 1;0 1 1 0 0 0;0 1 0 0 1 0;0 0 0 1 1 0]  CommutationSeqNeg="[0  1  1  0  0  0;0  1  0  0  1  0;0  0  0  1  1  0;1  0  0  1  0  0;1  0  0  0  0  1;0  0  1  0  0  1;]"
  switching3 : Outport
  wires:
  PositionInput/1 -> Six Step Commutation/1
  TorqueSign/1 -> Six Step Commutation/2
  Six Step Commutation/1 -> switching3/1  "switching"

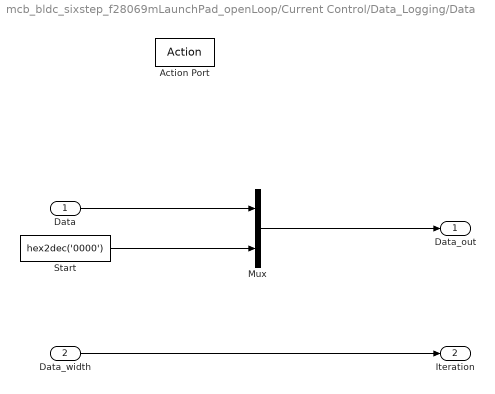
== system mcb_bldc_sixstep_f28069mLaunchPad_openLoop/Current Control/Data_Logging/Data ==
  Data : Inport
  Data_width : Inport  Port=2
  Action Port : ActionPort  ActionPortLabel=else
  Mux : Mux  Inputs=2
  Start : Constant  Value=hex2dec('0000')  OutDataTypeStr=uint16
  Data_out : Outport  VectorParamsAs1DForOutWhenUnconnected=off
  Iteration : Outport  Port=2  VectorParamsAs1DForOutWhenUnconnected=off
  wires:
  Start/1 -> Mux/2
  Mux/1 -> Data_out/1
  Data/1 -> Mux/1
  Data_width/1 -> Iteration/1

== system mcb_bldc_sixstep_f28069mLaunchPad_openLoop/Current Control/Data_Logging/Data_Conditioning ==
  In1 : Inport
  Data Type Conversion : DataTypeConversion  OutDataTypeStr=fixdt(1,16,12)  RndMeth=Simplest  SaturateOnIntegerOverflow=off
  Data Type Conversion1 : DataTypeConversion  OutDataTypeStr=uint16  ConvertRealWorld=Stored Integer (SI)  SaturateOnIntegerOverflow=off  RndMeth=Floor
  Out1 : Outport  VectorParamsAs1DForOutWhenUnconnected=off
  wires:
  In1/1 -> Data Type Conversion/1
  Data Type Conversion1/1 -> Out1/1
  Data Type Conversion/1 -> Data Type Conversion1/1

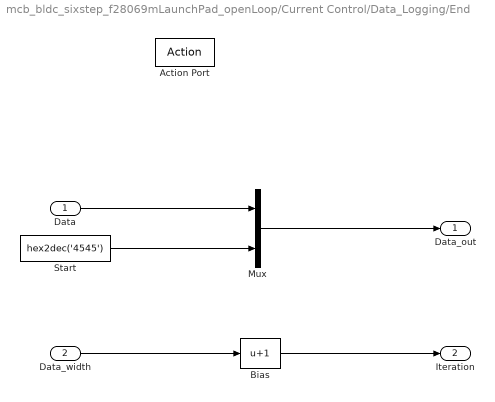
== system mcb_bldc_sixstep_f28069mLaunchPad_openLoop/Current Control/Data_Logging/End ==
  Data : Inport
  Data_width : Inport  Port=2
  Action Port : ActionPort  ActionPortLabel=elseif(u1 == 599)
  Bias : Bias  Bias=1  SaturateOnIntegerOverflow=off
  Mux : Mux  Inputs=2
  Start : Constant  Value=hex2dec('4545')  OutDataTypeStr=uint16
  Data_out : Outport  VectorParamsAs1DForOutWhenUnconnected=off
  Iteration : Outport  Port=2  VectorParamsAs1DForOutWhenUnconnected=off
  wires:
  Mux/1 -> Data_out/1
  Data_width/1 -> Bias/1
  Start/1 -> Mux/2
  Bias/1 -> Iteration/1
  Data/1 -> Mux/1

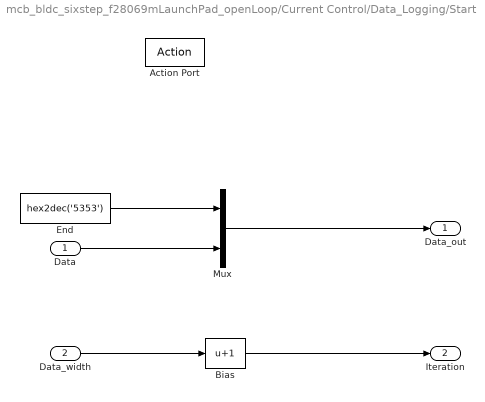
== system mcb_bldc_sixstep_f28069mLaunchPad_openLoop/Current Control/Data_Logging/Start ==
  Data : Inport
  Data_width : Inport  Port=2
  Action Port : ActionPort  ActionPortLabel=if(u1 == 0)
  Bias : Bias  Bias=1  SaturateOnIntegerOverflow=off
  End : Constant  Value=hex2dec('5353')  OutDataTypeStr=uint16
  Mux : Mux  Inputs=2
  Data_out : Outport  VectorParamsAs1DForOutWhenUnconnected=off
  Iteration : Outport  Port=2  VectorParamsAs1DForOutWhenUnconnected=off
  wires:
  End/1 -> Mux/1
  Mux/1 -> Data_out/1
  Data_width/1 -> Bias/1
  Bias/1 -> Iteration/1
  Data/1 -> Mux/2

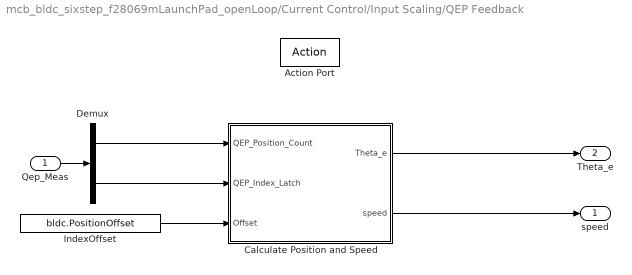
== system mcb_bldc_sixstep_f28069mLaunchPad_openLoop/Current Control/Input Scaling/QEP Feedback ==
  Qep_Meas : Inport
  Action Port : ActionPort  ActionPortLabel=if(u1 ==1)
  " Calculate Position and Speed" : Subsystem
  Demux : Demux  Outputs=2
  IndexOffset : Constant  Value=bldc.PositionOffset  OutDataTypeStr=dataType  SampleTime=-1
  speed : Outport
  Theta_e : Outport  Port=2
  wires:
  Demux/1 -> " Calculate Position and Speed"/1(QEP_Position_Count)
  IndexOffset/1 -> " Calculate Position and Speed"/3(Offset)
  Demux/2 -> " Calculate Position and Speed"/2(QEP_Index_Latch)
  " Calculate Position and Speed"/2(speed) -> speed/1
  " Calculate Position and Speed"/1(Theta_e) -> Theta_e/1
  Qep_Meas/1 -> Demux/1

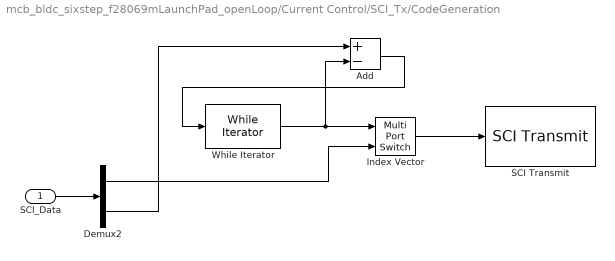
== system mcb_bldc_sixstep_f28069mLaunchPad_openLoop/Current Control/SCI_Tx/CodeGeneration ==
  SCI_Data : Inport
  Add : Sum  Inputs=+-  OutDataTypeStr=Inherit: Same as first input
  Demux2 : Demux  Outputs=2
  Index Vector : MultiPortSwitch  Inputs=1  SaturateOnIntegerOverflow=off  InputSameDT=off
  SCI Transmit : c280xlib/SCI Transmit  sciModule=A  dataHead=''  dataTail=''  frameSize=1  blockingMode=on  outputStatus=off
  While Iterator : WhileIterator  MaxIters=-1  WhileBlockType=do-while  ShowIterationPort=on  OutputDataType=int16
  wires:
  While Iterator/1 -> Index Vector/1, Add/2
  Demux2/1 -> Index Vector/2
  Index Vector/1 -> SCI Transmit/1
  Add/1 -> While Iterator/1
  Demux2/2 -> Add/1
  SCI_Data/1 -> Demux2/1

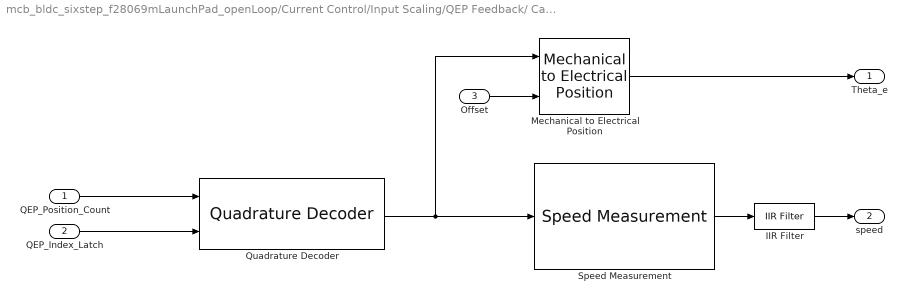
== system mcb_bldc_sixstep_f28069mLaunchPad_openLoop/Current Control/Input Scaling/QEP Feedback/ Calculate Position and Speed ==
  QEP_Position_Count : Inport
  QEP_Index_Latch : Inport  Port=2
  Offset : Inport  Port=3
  IIR Filter : mcbcontrolslib/IIR Filter  VariantControl=Low Pass Filter  VariantSelect=Low-pass  Filter_constant=0.01  advancedSettings=off  Ts=50e-6  cutOff_freq=32.1525
  Mechanical to Electrical Position : mcbpositiondecoderlib/Mechanical to Electrical Position  PolePairsInputType=Specify via dialog  NrPP=bldc.p  selectedRange=Per unit  MechOfstInputType=Input port  mechOffsetIn=0  maxAngleIn=1  InputDataType=dataType  VariantSelect=floating-point
  Quadrature Decoder : mcbpositiondecoderlib/Quadrature Decoder  EncoderSlitsPerRevolution=bldc.QEPSlits  EncoderCountsPerSlit=4  CounterSize=16 bits  ExternalIndexCount=on  PositionUnit=Per unit  PositionDataType=dataType  ParameterInputType=off  CountsPerRevInverseDataType=single
  Speed Measurement : mcbpositiondecoderlib/Speed Measurement  PositionUnit=Per unit  PositionScalingDatatype=uint32  SpeedCalculationMode=Time interval for speed calculation  SampleTimeAsync=Ts  MaximumApplicationSpeed=6000  SpeedResolution=5e-6  DelayLength=20  MaximumMeasurableSpeed=29999  MeasurableSpeedResolution=1.397e-05  SpeedUnit=Per unit based on dialog  PerUnitSpeed=PU_System.N_base  SpeedDataType=dataType
  Theta_e : Outport  VectorParamsAs1DForOutWhenUnconnected=off
  speed : Outport  Port=2  VectorParamsAs1DForOutWhenUnconnected=off
  wires:
  Speed Measurement/1 -> IIR Filter/1
  Mechanical to Electrical Position/1 -> Theta_e/1
  QEP_Position_Count/1 -> Quadrature Decoder/1
  Quadrature Decoder/1 -> Speed Measurement/1, Mechanical to Electrical Position/1
  Offset/1 -> Mechanical to Electrical Position/2
  IIR Filter/1 -> speed/1
  QEP_Index_Latch/1 -> Quadrature Decoder/2
